simulink model "ex3_sim2"  (R2018a)
settings: Solver=ode45  StartTime=0.0  StopTime=2  MaxStep=0.001  RelTol=1e-3  EnableMultiTasking=on
undefined symbols (not defined in the file): Ar, denP, DiscIntNeverNeededParam, kAWU, Kd, Ki, Kp, numP, t0r, TL, Ts
settings Model: Creator=antonello  LastModifiedBy=riccardo
settings DataIOCC: LimitDataPoints=on  SaveFormat=Array
settings OptimizationCC: LifeSpan=inf
settings DebuggingCC: SolverPrmCheckMsg=warning  SFUnexpectedBacktrackingDiag=warning  SFNoUnconditionalDefaultTransitionDiag=warning  SFExecutionAtInitializationDiag=none
settings HardwareCC: ProdBitPerPointer=32  ProdBitPerSizeT=32  ProdBitPerPtrDiffT=32  ProdLargestAtomicFloat=None  ProdIntDivRoundTo=Undefined  ProdEndianess=Unspecified  ProdWordSize=32  ProdHWDeviceType=32-bit Generic
settings ModelReferenceCC: PropagateSignalLabelsOutOfModel=off
settings CodeAppCC: StateflowObjectComments=on
settings GRTTargetCC: TargetLangStandard=C89/C90 (ANSI)  GeneratePreprocessorConditionals=Disable all
settings ConfigComp: CovMetricSettings=dw  CovHtmlReporting=on  CovSaveCumulativeToWorkspaceVar=on  CovSaveSingleToWorkspaceVar=on  CovExternalEMLEnable=off  CovSFcnEnable=off

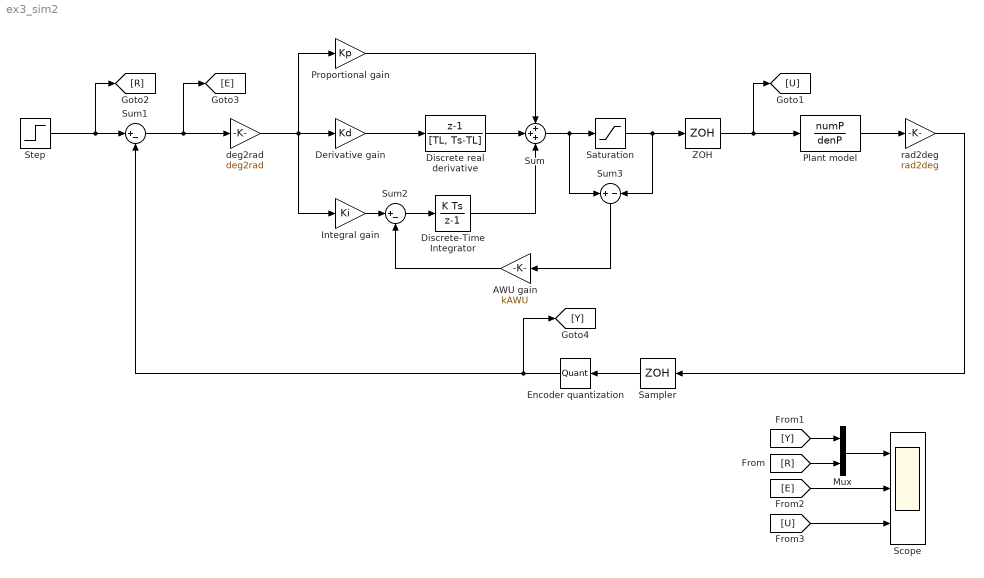
== system ex3_sim2 ==
  AWU gain : Gain  Gain=kAWU
  Derivative gain : Gain  Gain=Kd
  Discrete real derivative : DiscreteTransferFcn  Numerator=[1, -1]  Denominator=[TL, Ts-TL]  SampleTime=Ts
  Discrete-Time Integrator : DiscreteIntegrator  SampleTime=Ts  ICPrevOutput=DiscIntNeverNeededParam  ICPrevScaledInput=DiscIntNeverNeededParam
  Encoder quantization : Quantizer  QuantizationInterval=enc_pulse2deg
  Integral gain : Gain  Gain=Ki
  Mux : Mux  Inputs=2
  Plant model : TransferFcn  Numerator=numP  Denominator=denP
  Proportional gain : Gain  Gain=Kp
  Sampler : ZeroOrderHold  SampleTime=Ts
  Saturation : Saturate  UpperLimit=10  LowerLimit=-10
  Scope : Scope  NumInputPorts=3
  Step : Step  Time=t0r  After=Ar  SampleTime=Ts
  Sum : Sum  Inputs=+++
  Sum1 : Sum  Inputs=|+-
  Sum2 : Sum  Inputs=|+-
  Sum3 : Sum  Inputs=+-
  ZOH : ZeroOrderHold  SampleTime=Ts
  deg2rad : Gain  Gain=deg2rad
  rad2deg : Gain  Gain=rad2deg
  wires:
  Derivative gain/1 -> Discrete real derivative/1
  Proportional gain/1 -> Sum/1
  Sum1/1 -> [E], deg2rad/1
  Plant model/1 -> rad2deg/1
  Sum/1 -> Sum3/1, Saturation/1
  ZOH/1 -> Plant model/1, [U]
  Step/1 -> [R], Sum1/1
  Discrete real derivative/1 -> Sum/2
  Discrete-Time Integrator/1 -> Sum/3
  [Y] -> Mux/1
  [R] -> Mux/2
  Mux/1 -> Scope/1
  [E] -> Scope/2
  [U] -> Scope/3
  rad2deg/1 -> Sampler/1
  deg2rad/1 -> Integral gain/1, Derivative gain/1, Proportional gain/1
  Saturation/1 -> Sum3/2, ZOH/1
  Integral gain/1 -> Sum2/1
  Sum2/1 -> Discrete-Time Integrator/1
  Sum3/1 -> AWU gain/1
  AWU gain/1 -> Sum2/2
  Encoder quantization/1 -> [Y], Sum1/2
  Sampler/1 -> Encoder quantization/1
